simulink model "PDlev"  (R2015a)
settings: Solver=ode45  StartTime=0.0  StopTime=10.0  RelTol=1e-3
values from neighbouring files (symbols this model uses):
  g = 9.77    [TFLevitador.m]
  k = 7.5e-5    (= 7.5e-05)    [TFLevitador.m]
  L = 13.847e-3    (= 0.013847)    [TFLevitador.m]
  m = 5.85e-3    (= 0.00585)    [TFLevitador.m]
  R = 2.818    [TFLevitador.m]
undefined symbols (not defined in the file or in its folder): magnitude
libraries: simulink x1
settings Model: CovSFcnEnable=off  Creator=Daniel Tristan  LastModifiedBy=Oscar
settings OptimizationCC: BlockReduction=off  InlineParams=on  BufferReuse=off
settings DebuggingCC: SolverPrmCheckMsg=warning

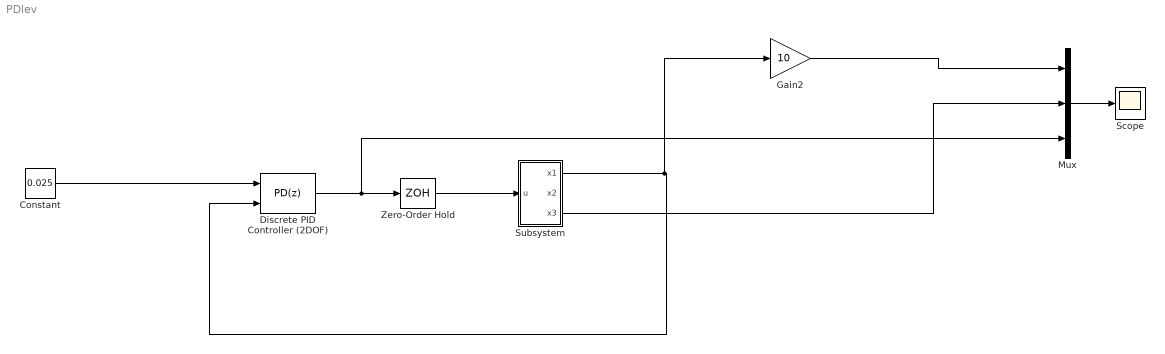
== system PDlev ==
  Constant : Constant  Value=0.025
  Discrete PID Controller (2DOF) : simulink/Continuous/PID Controller (2DOF)  Controller=PD  TimeDomain=Discrete-time  SampleTime=0.0010  IntegratorMethod=Forward Euler  FilterMethod=Forward Euler  Form=Parallel  UseFilter=on  ControllerParametersSource=internal  P=-383.15939214594  I=-115.550707260615  D=-22.9815666874815  N=685.016550997501  b=0.937120165899683  c=0.435867518843172  InitialConditionSource=internal  InitialConditionForIntegrator=0  InitialConditionForFilter=0  ExternalReset=none  LimitOutput=off  UpperSaturationLimit=inf  LowerSaturationLimit=-inf  LinearizeAsGain=off  AntiWindupMode=none  Kb=1  TrackingMode=off  Kt=1  PParamMin=[]  PParamMax=[]  IParamMin=[]  IParamMax=[]  DParamMin=[]  DParamMax=[]  NParamMin=[]  NParamMax=[]  bParamMin=[]  bParamMax=[]  cParamMin=[]  cParamMax=[]  KbParamMin=[]  KbParamMax=[]  KtParamMin=[]  KtParamMax=[]  POutMin=[]  POutMax=[]  IOutMin=[]  IOutMax=[]  DOutMin=[]  DOutMax=[]  NOutMin=[]  NOutMax=[]  bOutMin=[]  bOutMax=[]  cOutMin=[]  cOutMax=[]  KbOutMin=[]  KbOutMax=[]  KtOutMin=[]  KtOutMax=[]  IntegratorOutMin=[]  IntegratorOutMax=[]  FilterOutMin=[]  FilterOutMax=[]  SumOutMin=[]  SumOutMax=[]  Sum1OutMin=[]  Sum1OutMax=[]  Sum2OutMin=[]  Sum2OutMax=[]  Sum3OutMin=[]  Sum3OutMax=[]  SumI1OutMin=[]  SumI1OutMax=[]  SumI2OutMin=[]  SumI2OutMax=[]  SumI3OutMin=[]  SumI3OutMax=[]  SumDOutMin=[]  SumDOutMax=[]  SaturationOutMin=[]  SaturationOutMax=[]  IntegratorContinuousStateAttributes=''  IntegratorStateMustResolveToSignalObject=off  IntegratorRTWStateStorageClass=Auto  FilterContinuousStateAttributes=''  FilterStateMustResolveToSignalObject=off  FilterRTWStateStorageClass=Auto  DifferentiatorICPrevScaledInput=0  DifferentiatorOutMin=[]  DifferentiatorOutMax=[]
  Gain2 : Gain  Gain=10
  Mux : Mux  Inputs=3
  Scope : Scope
      settings: TimeRange=10  YMin=-100  YMax=500
  Subsystem : Subsystem
  Zero-Order Hold : ZeroOrderHold  SampleTime=0.001
  wires:
  Constant/1 -> Discrete PID Controller (2DOF)/1
  Mux/1 -> Scope/1
  Discrete PID Controller (2DOF)/1 -> Mux/3, Zero-Order Hold/1
  Zero-Order Hold/1 -> Subsystem/1(u)
  Subsystem/1(x1) -> Gain2/1, Discrete PID Controller (2DOF)/2
  Gain2/1 -> Mux/1
  Subsystem/3(x3) -> Mux/2

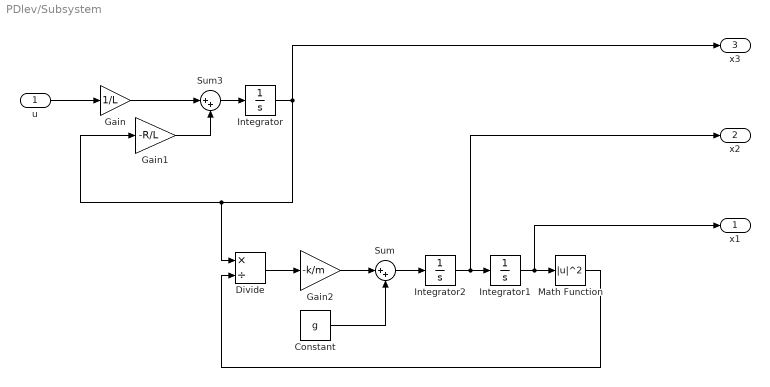
== system PDlev/Subsystem ==
  u : Inport
  Constant : Constant  Value=g
  Divide : Product  Inputs=*/
  Gain : Gain  Gain=1/L
  Gain1 : Gain  Gain=-R/L
  Gain2 : Gain  Gain=-k/m
  Integrator : Integrator  InitialCondition=0.06  UpperSaturationLimit=1  LowerSaturationLimit=0
  Integrator1 : Integrator  InitialCondition=0.05  UpperSaturationLimit=1  LowerSaturationLimit=0
  Integrator2 : Integrator
  Math Function : Math  Operator=magnitude^2  SaturateOnIntegerOverflow=on
  Sum : Sum  Inputs=|++
  Sum3 : Sum  Inputs=|++
  x1 : Outport
  x2 : Outport  Port=2
  x3 : Outport  Port=3
  wires:
  Gain2/1 -> Sum/1
  Integrator1/1 -> x1/1, Math Function/1
  Integrator2/1 -> x2/1, Integrator1/1
  Constant/1 -> Sum/2
  Sum3/1 -> Integrator/1
  Integrator/1 -> Divide/1, Gain1/1, x3/1
  Gain1/1 -> Sum3/2
  Sum/1 -> Integrator2/1
  Divide/1 -> Gain2/1
  Math Function/1 -> Divide/2
  u/1 -> Gain/1
  Gain/1 -> Sum3/1
